simulink model "Autopilot_mdl_pcss"  (R2018b)
settings: Solver=VariableStepAuto  StartTime=0.0  StopTime=1  MaxStep=0.01  RelTol=1e-3  EnableMultiTasking=on
libraries: lpvlibrary x4, simulink x1
settings Model: Creator=Fernando  LastModifiedBy=ferna
settings OptimizationCC: LifeSpan=inf
settings DebuggingCC: SFUnexpectedBacktrackingDiag=warning  SFNoUnconditionalDefaultTransitionDiag=warning
settings SFSimCC: SimUseLocalCustomCode=off
settings RTWCC: RTWUseLocalCustomCode=off
settings CodeAppCC: StateflowObjectComments=on
settings GRTTargetCC: TargetLangStandard=C89/C90 (ANSI)  GeneratePreprocessorConditionals=Disable all
settings ConfigComp: CovMetricSettings=dw  CovHtmlReporting=on  CovSaveCumulativeToWorkspaceVar=on  CovSaveSingleToWorkspaceVar=on  CovExternalEMLEnable=off

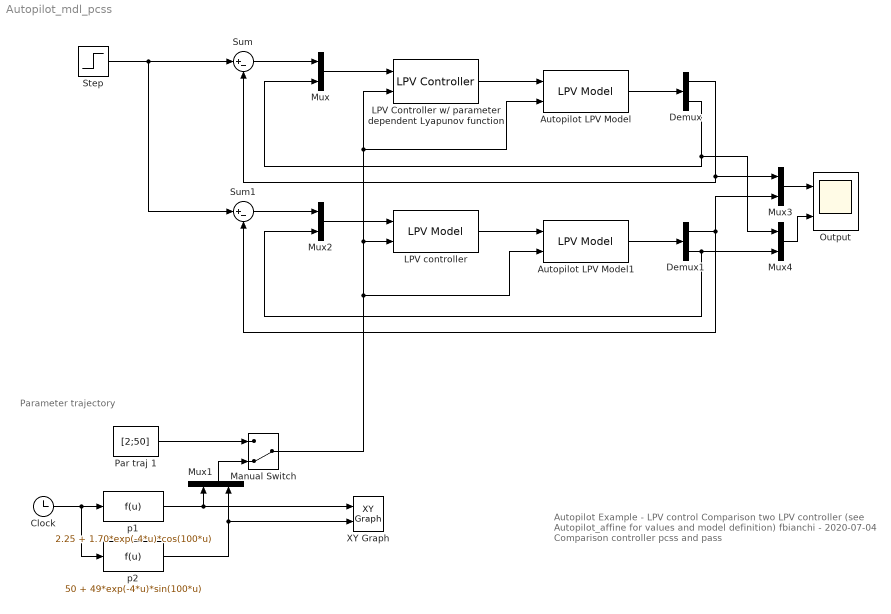
== system Autopilot_mdl_pcss ==
  note: Autopilot Example - LPV control
      | Comparison two LPV controller
      | (see Autopilot_affine for values and model definition)
      | fbianchi - 2020-07-04
      | Comparison controller pcss and pass
  note: Parameter trajectory
  Autopilot LPV Model : lpvlibrary/LPV Model  pdSys=pdG  x0=0
      settings: SourceProductName=LPV Toolbox
  Autopilot LPV Model1 : lpvlibrary/LPV Model  pdSys=pdG  x0=0
      settings: SourceProductName=LPV Toolbox
  Clock : Clock
  Demux : Demux  Outputs=2
  Demux1 : Demux  Outputs=2
  LPV Controller w/ parameter dependent Lyapunov function : lpvlibrary/LPV Controller  pdSys=pdK3  x0=0
      settings: SourceProductName=LPV Toolbox
  LPV controller : lpvlibrary/LPV Model  pdSys=pdK2  x0=0
      settings: SourceProductName=LPV Toolbox
  Manual Switch : ManualSwitch  CurrentSetting=0
  Mux{,1..4} (5 alike) : Mux  Inputs=2
  Output : Scope  NumInputPorts=2
  Par traj 1 : Constant  Value=[2;50]
  Step : Step  Time=0.2  SampleTime=0
  Sum : Sum  Inputs=|+-
  Sum1 : Sum  Inputs=|+-
  XY Graph : simulink/Sinks/XY Graph  xmin=0  xmax=5  ymin=0  ymax=110  st=-1
  p1 : Fcn  Expr=2.25 + 1.70*exp(-4*u)*cos(100*u)
  p2 : Fcn  Expr=50 + 49*exp(-4*u)*sin(100*u)
  wires:
  Autopilot LPV Model/1 -> Demux/1
  Demux/1 -> Mux3/1, Sum/2
  Demux/2 -> Mux4/1, Mux/2
  LPV Controller w/ parameter dependent Lyapunov function/1 -> Autopilot LPV Model/1
  Mux/1 -> LPV Controller w/ parameter dependent Lyapunov function/1
  Sum/1 -> Mux/1
  Clock/1 -> p2/1, p1/1
  p1/1 -> Mux1/1, XY Graph/1
  p2/1 -> XY Graph/2, Mux1/2
  Mux1/1 -> Manual Switch/2
  Par traj 1/1 -> Manual Switch/1
  Manual Switch/1 -> Autopilot LPV Model1/2, LPV controller/2, LPV Controller w/ parameter dependent Lyapunov function/2, Autopilot LPV Model/2
  Autopilot LPV Model1/1 -> Demux1/1
  Demux1/1 -> Sum1/2, Mux3/2
  Demux1/2 -> Mux2/2, Mux4/2
  LPV controller/1 -> Autopilot LPV Model1/1
  Step/1 -> Sum1/1, Sum/1
  Mux2/1 -> LPV controller/1
  Sum1/1 -> Mux2/1
  Mux3/1 -> Output/1
  Mux4/1 -> Output/2
